simulink model "ThreephaseInverterTrialOut"  (R2016a)
settings: Solver=FixedStepAuto  StartTime=0.5  StopTime=1  FixedStep=0.0001  RelTol=1  AbsTol=0.1
libraries: nesl_utility x10, pe_lib x6, elec_lib x4, fl_lib x4, powerlib_meascontrol x1
settings Model: Creator=syf  LastModifiedBy=syf

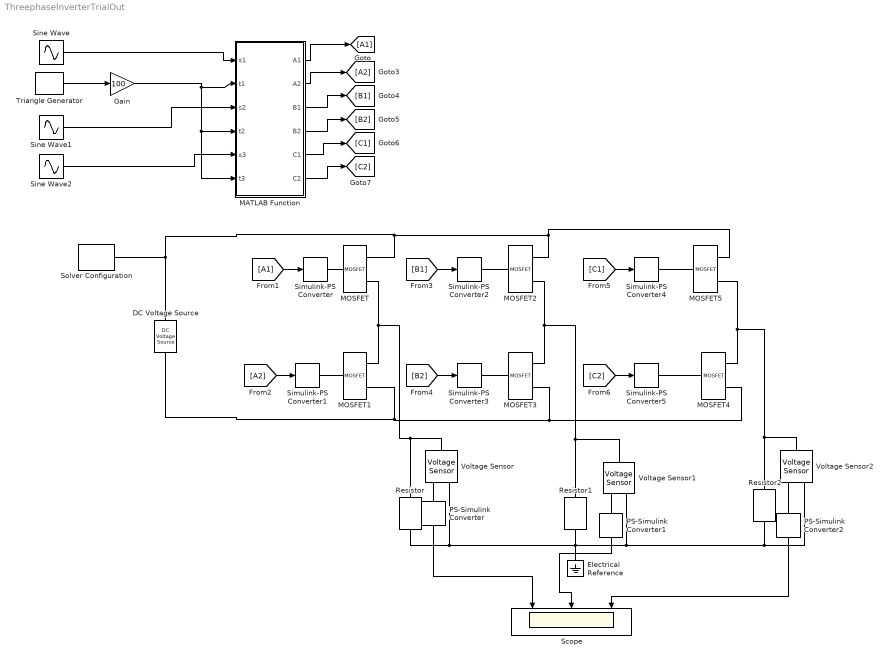
== system ThreephaseInverterTrialOut ==
  DC Voltage Source : elec_lib/Additional Components/SPICE-Compatible Components/Sources/DC Voltage Source  DC=100 V
  Electrical Reference : fl_lib/Electrical/Electrical Elements/Electrical Reference
  Gain : Gain  Gain=100
  MATLAB Function : MATLAB Function  TreatAsAtomicUnit=on
  MOSFET{,1..5} (6 alike) : pe_lib/Semiconductors/Fundamental Components/MOSFET  Rds=0.01 Ohm  Goff=1e-6 1/Ohm  Vth=2 V  diode_param=2  diode_Vf=0.8 V  diode_Ron=0.001 Ohm  diode_Goff=1e-5 1/Ohm  diode_C=5e-8 F  diode_iRM=-235 A  diode_iF=300 A  diode_idot=-50 A/us  diode_trr_param=1  diode_trr_factor=3  diode_trr=15 us  diode_Qrr=1.5e+3 s*uA
  PS-Simulink Converter : nesl_utility/PS-Simulink Converter  PhysicalDomain=network_engine_domain  SubClassName=ps_output  LeftPortType=input  RightPortType=output  PseudoPeriodic=off  Frequencies=[]  Unit=1  AffineConversion=off
  PS-Simulink Converter1 : nesl_utility/PS-Simulink Converter  PhysicalDomain=network_engine_domain  SubClassName=ps_output  LeftPortType=input  RightPortType=output  PseudoPeriodic=off  Frequencies=[]  Unit=1  AffineConversion=off
  PS-Simulink Converter2 : nesl_utility/PS-Simulink Converter  PhysicalDomain=network_engine_domain  SubClassName=ps_output  LeftPortType=input  RightPortType=output  PseudoPeriodic=off  Frequencies=[]  Unit=1  AffineConversion=off
  Resistor : elec_lib/Passive Devices/Resistor  R=1 Ohm  R_tol=5  enable_R_tol=0  tol_distribution=1  nSigma=4  enable_operating_limits=0  operating_limit_action=2  max_working_voltage=100 V  power_rating=1 W  enable_faults=0  fault_action=1  R_faulted=Inf Ohm  enable_temporal_fault=0  t_fault=1 s  enable_behavioral_fault=0  max_permissible_current=1 A  t_fail_on_current=1 s  noise_mode=0  sample_time=0.001 s  repeatability=1  auto_seed=2843309574  user_seed=0  Tdevice=25 degC  alpha=0.00393 1/K  Tmeas=25 degC  thermal_mass=100 J/K  initial_temperature=25 degC  power_derating_T1=70 degC  power_derating_T2=155 degC  operating_temperature_range_vec=[ -50 150 ] degC
  Resistor1 : elec_lib/Passive Devices/Resistor  R=1 Ohm  R_tol=5  enable_R_tol=0  tol_distribution=1  nSigma=4  enable_operating_limits=0  operating_limit_action=2  max_working_voltage=100 V  power_rating=1 W  enable_faults=0  fault_action=1  R_faulted=Inf Ohm  enable_temporal_fault=0  t_fault=1 s  enable_behavioral_fault=0  max_permissible_current=1 A  t_fail_on_current=1 s  noise_mode=0  sample_time=0.001 s  repeatability=1  auto_seed=1846498393  user_seed=0  Tdevice=25 degC  alpha=0.00393 1/K  Tmeas=25 degC  thermal_mass=100 J/K  initial_temperature=25 degC  power_derating_T1=70 degC  power_derating_T2=155 degC  operating_temperature_range_vec=[ -50 150 ] degC
  Resistor2 : elec_lib/Passive Devices/Resistor  R=1 Ohm  R_tol=5  enable_R_tol=0  tol_distribution=1  nSigma=4  enable_operating_limits=0  operating_limit_action=2  max_working_voltage=100 V  power_rating=1 W  enable_faults=0  fault_action=1  R_faulted=Inf Ohm  enable_temporal_fault=0  t_fault=1 s  enable_behavioral_fault=0  max_permissible_current=1 A  t_fail_on_current=1 s  noise_mode=0  sample_time=0.001 s  repeatability=1  auto_seed=3812947214  user_seed=0  Tdevice=25 degC  alpha=0.00393 1/K  Tmeas=25 degC  thermal_mass=100 J/K  initial_temperature=25 degC  power_derating_T1=70 degC  power_derating_T2=155 degC  operating_temperature_range_vec=[ -50 150 ] degC
  Scope : Scope  NumInputPorts=3
  Simulink-PS Converter{,1..5} (6 alike) : nesl_utility/Simulink-PS Converter  PhysicalDomain=network_engine_domain  SubClassName=ps_input  LeftPortType=input  RightPortType=output  PseudoPeriodic=off  Frequencies=[]  NoiseDistribution=none  NoiseParameters=[]  Unit=1  AffineConversion=off  InputFiltering=off  SimscapeFilterOrder=1  InputFilterTimeConstant=0.001  UdotUserProvided=1
  Sine Wave : Sin  Amplitude=80  Frequency=100*pi  SampleTime=0
  Sine Wave1 : Sin  Amplitude=80  Frequency=100*pi  Phase=2/3*pi  SampleTime=0
  Sine Wave2 : Sin  Amplitude=80  Frequency=100*pi  Phase=-2/3*pi  SampleTime=0
  Solver Configuration : nesl_utility/Solver Configuration  PhysicalDomain=network_engine_domain  SubClassName=solver  LeftPortType=input  RightPortType=generic  Accelerate=off  Tones=[]  Harmonics=[]  SimulateNoise=off  Profile=off  UseLocalSampling=off  EnableSwitchedLinearOptims=on  FrequencyDomain=off  UseCCode=off  RelTol=0.001  AbsTol=1e-06  MinStep=1e-09  ToWorkspace=off  RevertToSquareIcSolve=off  NumHomotopyIterations=100  PhasorMode=off  PhasorModeNumHarmonics=1  OverrideAbsTol=off  DoDC=off  ResidualTolerance=1e-10  UseLocalSolver=off  LocalSolverChoice=NE_BACKWARD_EULER_ADVANCER  LocalSolverSampleTime=0.001  DoFixedCost=off  MaxNonlinIter=3  MaxModeIter=2  LinearAlgebra=Sparse  DelaysMemoryBudget=1024  AutomaticFiltering=on  FilteringTimeConstant=0.001
  Triangle Generator : powerlib_meascontrol/Pulse & Signal Generators/Triangle Generator  Freq=100  Phase=90  Ts=0
  Voltage Sensor : fl_lib/Electrical/Electrical Sensors/Voltage Sensor
  Voltage Sensor1 : fl_lib/Electrical/Electrical Sensors/Voltage Sensor
  Voltage Sensor2 : fl_lib/Electrical/Electrical Sensors/Voltage Sensor
  wires:
  Triangle Generator/1 -> Gain/1
  Sine Wave/1 -> MATLAB Function/1(s1)
  Gain/1 -> MATLAB Function/2(t1), MATLAB Function/6(t3), MATLAB Function/4(t2)
  MATLAB Function/1(A1) -> [A1]
  Sine Wave1/1 -> MATLAB Function/3(s2)
  Sine Wave2/1 -> MATLAB Function/5(s3)
  MATLAB Function/2(A2) -> [A2]
  MATLAB Function/3(B1) -> [B1]
  MATLAB Function/4(B2) -> [B2]
  MATLAB Function/5(C1) -> [C1]
  MATLAB Function/6(C2) -> [C2]
  [A1] -> Simulink-PS Converter/1
  [A2] -> Simulink-PS Converter1/1
  [B1] -> Simulink-PS Converter2/1
  [B2] -> Simulink-PS Converter3/1
  [C1] -> Simulink-PS Converter4/1
  [C2] -> Simulink-PS Converter5/1
  PS-Simulink Converter/1 -> Scope/1
  PS-Simulink Converter1/1 -> Scope/2
  PS-Simulink Converter2/1 -> Scope/3
  connections:
  MOSFET/RConn2 -- MOSFET1/RConn1 -- Voltage Sensor/LConn1 -- Resistor/LConn1
  MOSFET2/RConn2 -- Voltage Sensor1/LConn1 -- Resistor1/LConn1 -- MOSFET3/RConn1
  MOSFET5/RConn2 -- Voltage Sensor2/LConn1 -- Resistor2/LConn1 -- MOSFET4/RConn1
  Solver Configuration/RConn1 -- DC Voltage Source/LConn1 -- MOSFET2/RConn1 -- MOSFET5/RConn1 -- MOSFET/RConn1
  MOSFET3/RConn2 -- MOSFET4/RConn2 -- DC Voltage Source/RConn1 -- MOSFET1/RConn2
  Simulink-PS Converter/RConn1 -- MOSFET/LConn1
  Simulink-PS Converter1/RConn1 -- MOSFET1/LConn1
  Simulink-PS Converter2/RConn1 -- MOSFET2/LConn1
  Simulink-PS Converter3/RConn1 -- MOSFET3/LConn1
  Simulink-PS Converter4/RConn1 -- MOSFET5/LConn1
  Simulink-PS Converter5/RConn1 -- MOSFET4/LConn1
  Resistor/RConn1 -- Electrical Reference/LConn1 -- Voltage Sensor1/RConn2 -- Voltage Sensor2/RConn2 -- Resistor2/RConn1 -- Resistor1/RConn1 -- Voltage Sensor/RConn2
  PS-Simulink Converter/LConn1 -- Voltage Sensor/RConn1
  PS-Simulink Converter1/LConn1 -- Voltage Sensor1/RConn1
  PS-Simulink Converter2/LConn1 -- Voltage Sensor2/RConn1

== matlab function ThreephaseInverterTrialOut/MATLAB Function ==
  data: s1 input; A1 output; t1 input; A2 output; s2 input; t2 input; s3 input; t3 input; B1 output; B2 output; C1 output; C2 output
function [A1, A2, B1, B2,C1, C2] = fcn(s1,t1,s2,t2,s3,t3)
    if s1<t1 
        A1=6;
        A2=0;
    else 
        A1=0;
        A2=6;
    end
    
    if s2<t2
        B1=6;
        B2=0;
    else 
        B1=0;
        B2=6;
    end
    
    if s3<t3
        C1=6;
        C2=0;
    else 
        C1=0;
        C2=6;
    end
